simulink model "MoWiTO_mpc_FAST"  (Simulink 10.0)
settings: Solver=ode4  StartTime=0.0  StopTime=TMax  FixedStep=DT  MaxStep=DT  RelTol=1e-3  EnableMultiTasking=on
undefined symbols (not defined in the file or in its folder): beta_min, DiscIntNeverNeededParam, DT_control, DT_hw, FBonly, mpc, N, N_delay, N_filt, Nominal, OutList, strmatch, TurbParams
libraries: dspbuff3 x1
settings Model: Creator=bjonkman  LastModifiedBy=tskib
settings DataIOCC: LimitDataPoints=on  SignalLoggingSaveFormat=ModelDataLogs  SaveOutput=off  SaveTime=off  SignalLoggingName=sigsOut
settings OptimizationCC: ExpressionDepthLimit=2147483647
settings DebuggingCC: SaveWithParameterizedLinksMsg=none  SignalResolutionControl=TryResolveAllWithWarning  MultiTaskDSMMsg=warning  MultiTaskCondExecSysMsg=none  FcnCallInpInsideContextMsg=warning  AllowSymbolicDim=off  StateNameClashWarn=warning
settings HardwareCC: TargetUnknown=on
settings GRTTargetCC: GeneratePreprocessorConditionals=Disable all
settings ConfigComp: CovExternalEMLEnable=off

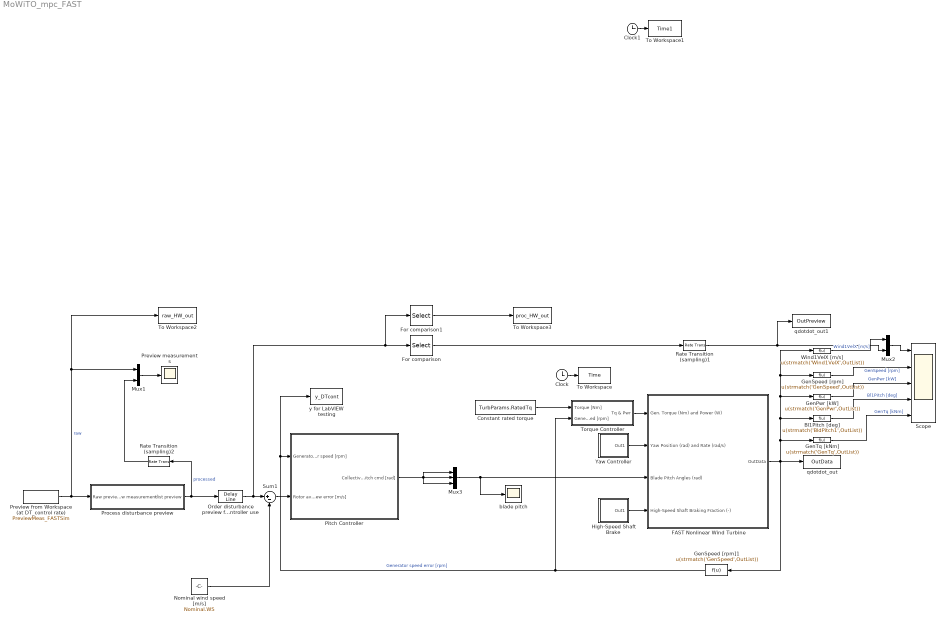
== system MoWiTO_mpc_FAST ==
  Bl1Pitch [deg] : Fcn  Expr=u(strmatch('BldPitch1',OutList))
  Clock : Clock
  Clock1 : Clock
  Constant rated torque : Constant  Value=TurbParams.RatedTq
  FAST Nonlinear Wind Turbine : Subsystem  mask(FAST Nonlinear Wind Turbine){}
      mask help: This block contains the FAST S-Function.
      mask init:
      | clear FAST_SFunc
  For comparison : Selector  InputPortWidth=N  IndexOptions=Index vector (dialog)  Indices=[1]  OutputSizes=1
  For comparison1 : Selector  InputPortWidth=N  IndexOptions=Index vector (dialog)  Indices=[N]  OutputSizes=1
  GenPwr [kW] : Fcn  Expr=u(strmatch('GenPwr',OutList))
  GenSpeed [rpm] : Fcn  Expr=u(strmatch('GenSpeed',OutList))
  GenSpeed [rpm]1 : Fcn  Expr=u(strmatch('GenSpeed',OutList))
  GenTq [kNm] : Fcn  Expr=u(strmatch('GenTq',OutList))
  High-Speed Shaft Brake : Subsystem
  Mux1 : Mux  Inputs=2
  Mux2 : Mux  Inputs=2
  Mux3 : Mux  Inputs=3
  Nominal wind speed [m/s] : Constant  Value=Nominal.WS
  Order disturbance preview for controller use : dspbuff3/Delay Line  siz=N  ic=Nominal.WS  directfeed=off  enable_output=off  hold_output=off  OutputFrames=off
      settings: SourceProductName=DSP System Toolbox  SourceProductBaseCode=DS
  Pitch Controller : Subsystem
  Preview from Workspace (at DT_control rate) : FromWorkspace  VariableName=PreviewMeas_FASTSim  SampleTime=DT_hw
  Preview measurements : Scope
  Process disturbance preview : Subsystem
  Rate Transition (sampling)1 : RateTransition  InitialCondition=Nominal.WS  OutPortSampleTime=DT
  Rate Transition (sampling)2 : RateTransition  OutPortSampleTime=DT_hw
  Scope : Scope  NumInputPorts=5
  Sum1 : Sum  Inputs=|+-
  To Workspace : ToWorkspace  VariableName=Time  SampleTime=-1
  To Workspace1 : ToWorkspace  VariableName=Time1  SampleTime=-1
  To Workspace2 : ToWorkspace  VariableName=raw_HW_out  SampleTime=-1
  To Workspace3 : ToWorkspace  VariableName=proc_HW_out  SampleTime=-1
  Torque Controller : Subsystem
  Wind1VelX [m/s] : Fcn  Expr=u(strmatch('Wind1VelX',OutList))
  Yaw Controller : Subsystem
  blade pitch : Scope
  qdotdot_out : ToWorkspace  VariableName=OutData  SampleTime=-1
  qdotdot_out1 : ToWorkspace  VariableName=OutPreview  SampleTime=-1
  y for LabVIEW testing : ToWorkspace  VariableName=y_DTcont  SampleTime=-1
  wires:
  Clock/1 -> To Workspace/1
  FAST Nonlinear Wind Turbine/1(OutData) -> GenSpeed [rpm]1/1, GenTq [kNm]/1, Bl1Pitch [deg]/1, GenPwr [kW]/1, GenSpeed [rpm]/1, Wind1VelX [m/s]/1, qdotdot_out/1
  Torque Controller/1(Tq & Pwr) -> FAST Nonlinear Wind Turbine/1(Gen. Torque (Nm) and Power (W))
  Yaw Controller/1(Out1) -> FAST Nonlinear Wind Turbine/2(Yaw Position (rad) and Rate (rad/s))
  Mux3/1 -> FAST Nonlinear Wind Turbine/3(Blade Pitch Angles (rad)), blade pitch/1
  High-Speed Shaft Brake/1(Out1) -> FAST Nonlinear Wind Turbine/4(High-Speed Shaft Braking Fraction (-))
  Constant rated torque/1 -> Torque Controller/1(Torque [Nm])
  Wind1VelX [m/s]/1 -> Mux2/1  "Wind1VelX [m/s]"
  GenSpeed [rpm]/1 -> Scope/2  "GenSpeed [rpm]"
  GenPwr [kW]/1 -> Scope/3  "GenPwr [kW]"
  Bl1Pitch [deg]/1 -> Scope/4  "Bl1Pitch [deg]"
  GenTq [kNm]/1 -> Scope/5  "GenTq [kNm]"
  GenSpeed [rpm]1/1 -> y for LabVIEW testing/1, Pitch Controller/1("Generator speed [rpm] "), Torque Controller/2(Generator speed [rpm])  "Generator speed error [rpm]"
  Process disturbance preview/1(dist preview) -> Order disturbance preview for controller use/1, Rate Transition (sampling)2/1  "processed"
  Clock1/1 -> To Workspace1/1
  Sum1/1 -> Pitch Controller/2(Rotor average speed preview error [m/s])
  Nominal wind speed [m/s]/1 -> Sum1/2
  Mux1/1 -> Preview measurements/1
  Preview from Workspace (at DT_control rate)/1 -> Process disturbance preview/1(Raw preview measurement), To Workspace2/1, Mux1/1  "raw"
  Mux2/1 -> Scope/1
  For comparison/1 -> Rate Transition (sampling)1/1
  Rate Transition (sampling)2/1 -> Mux1/2
  Rate Transition (sampling)1/1 -> qdotdot_out1/1, Mux2/2
  Pitch Controller/1(Collective pitch cmd [rad]) -> Mux3/3, Mux3/1, Mux3/2
  For comparison1/1 -> To Workspace3/1
  Order disturbance preview for controller use/1 -> For comparison1/1, For comparison/1, Sum1/1

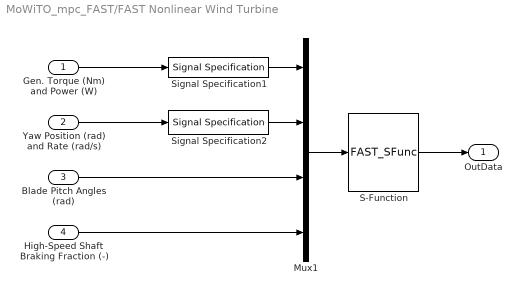
== system MoWiTO_mpc_FAST/FAST Nonlinear Wind Turbine ==
  Gen. Torque (Nm) and Power (W) : Inport
  Yaw Position (rad) and Rate (rad/s) : Inport  Port=2
  Blade Pitch Angles (rad) : Inport  Port=3
  High-Speed Shaft Braking Fraction (-) : Inport  Port=4
  Mux1 : Mux
  S-Function : S-Function  FunctionName=FAST_SFunc  Parameters=FAST_InputFileName, TMax, 0  SFunctionDeploymentMode=off  EnableBusSupport=off
  Signal Specification1 : SignalSpecification  OutDataTypeStr=double  Dimensions=2
  Signal Specification2 : SignalSpecification  OutDataTypeStr=double  Dimensions=2
  OutData : Outport
  wires:
  Gen. Torque (Nm) and Power (W)/1 -> Signal Specification1/1
  S-Function/1 -> OutData/1
  Mux1/1 -> S-Function/1
  Blade Pitch Angles (rad)/1 -> Mux1/3
  Yaw Position (rad) and Rate (rad/s)/1 -> Signal Specification2/1
  Signal Specification1/1 -> Mux1/1
  Signal Specification2/1 -> Mux1/2
  High-Speed Shaft Braking Fraction (-)/1 -> Mux1/4

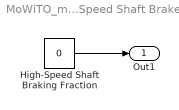
== system MoWiTO_mpc_FAST/High-Speed Shaft Brake ==
  High-Speed Shaft Braking Fraction : Constant  Value=0
  Out1 : Outport
  wires:
  High-Speed Shaft Braking Fraction/1 -> Out1/1

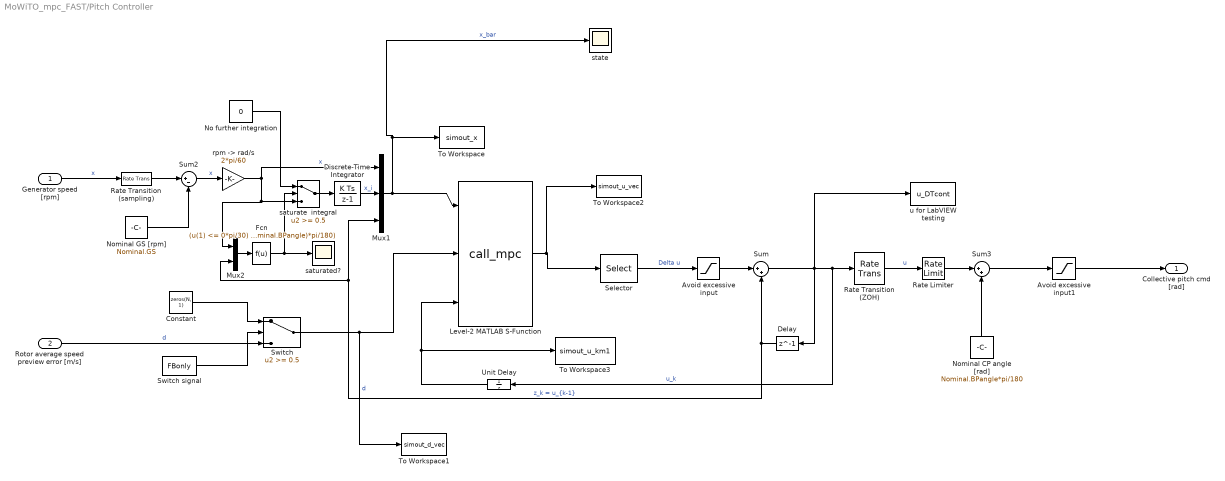
== system MoWiTO_mpc_FAST/Pitch Controller ==
  "Generator speed [rpm] " : Inport
  Rotor average speed preview error [m/s] : Inport  Port=2
  Avoid excessive input : Saturate  UpperLimit=TurbParams.PitchRateLimit*DT_control  LowerLimit=-TurbParams.PitchRateLimit*DT_control
  Avoid excessive input1 : Saturate  UpperLimit=inf  LowerLimit=beta_min*pi/180
  Constant : Constant  Value=zeros(N, 1)
  Delay : Delay  DelayLength=1  InitialCondition=0  SampleTime=DT_control
  Discrete-Time Integrator : DiscreteIntegrator  SampleTime=DT_control  ICPrevOutput=DiscIntNeverNeededParam  ICPrevScaledInput=DiscIntNeverNeededParam
  Fcn : Fcn  Expr=(u(1) <= 0*pi/30) && (u(2) <= (beta_min - Nominal.BPangle)*pi/180)
  Level-2 MATLAB S-Function : M-S-Function  FunctionName=call_mpc  Parameters=mpc
  Mux1 : Mux  Inputs=3
  Mux2 : Mux  Inputs=2
  No further integration : Constant  Value=0
  Nominal CP angle [rad] : Constant  Value=Nominal.BPangle*pi/180
  Nominal GS [rpm] : Constant  Value=Nominal.GS
  Rate Limiter : RateLimiter  RisingSlewLimit=TurbParams.PitchRateLimit  FallingSlewLimit=-TurbParams.PitchRateLimit  SampleTimeMode=inherited
  Rate Transition (ZOH) : RateTransition  OutPortSampleTime=DT
  Rate Transition (sampling) : RateTransition  OutPortSampleTime=DT_control
  Selector : Selector  InputPortWidth=mpc.Mdl.m*mpc.N  IndexOptions=Index vector (dialog)  Indices=[1:mpc.Mdl.m]  OutputSizes=1
  Sum : Sum  Inputs=|++  OutDataTypeStr=Inherit: Inherit via back propagation
  Sum2 : Sum  Inputs=|+-
  Sum3 : Sum  Inputs=|++
  Switch : Switch  Threshold=0.5
  Switch signal : Constant  Value=FBonly
  To Workspace : ToWorkspace  VariableName=simout_x  SampleTime=-1
  To Workspace1 : ToWorkspace  VariableName=simout_d_vec  SampleTime=-1
  To Workspace2 : ToWorkspace  VariableName=simout_u_vec  SampleTime=-1
  To Workspace3 : ToWorkspace  VariableName=simout_u_km1  SampleTime=-1
  Unit Delay : UnitDelay  SampleTime=DT_control  HasFrameUpgradeWarning=on
  "rpm -> rad/s" : Gain  Gain=2*pi/60
  saturate  integral : Switch  Threshold=0.5
  saturated? : Scope
  state : Scope
  u for LabVIEW testing : ToWorkspace  VariableName=u_DTcont  SampleTime=-1
  Collective pitch cmd [rad] : Outport
  wires:
  Delay/1 -> Mux1/3, Mux2/2, Sum/2  "z_k = u_{k-1}"
  Sum/1 -> u for LabVIEW testing/1, Unit Delay/1, Rate Transition (ZOH)/1, Delay/1  "u_k"
  Selector/1 -> Avoid excessive input/1  "Delta u"
  Rotor average speed preview error [m/s]/1 -> Switch/3  "d"
  "rpm -> rad/s"/1 -> Mux2/1, saturate  integral/3, Mux1/1  "x"
  Discrete-Time Integrator/1 -> Mux1/2  "x_i"
  Sum2/1 -> "rpm -> rad/s"/1  "x"
  Mux1/1 -> state/1, To Workspace/1, Level-2 MATLAB S-Function/1  "x_bar"
  Avoid excessive input/1 -> Sum/1
  Nominal GS [rpm]/1 -> Sum2/2
  "Generator speed [rpm] "/1 -> Rate Transition (sampling)/1  "x"
  Rate Transition (sampling)/1 -> Sum2/1
  Nominal CP angle [rad]/1 -> Sum3/2
  Rate Limiter/1 -> Sum3/1
  Rate Transition (ZOH)/1 -> Rate Limiter/1  "u"
  Switch signal/1 -> Switch/2
  Level-2 MATLAB S-Function/1 -> To Workspace2/1, Selector/1
  Sum3/1 -> Avoid excessive input1/1
  Unit Delay/1 -> Level-2 MATLAB S-Function/3, To Workspace3/1
  Switch/1 -> Level-2 MATLAB S-Function/2, To Workspace1/1  "d"
  Constant/1 -> Switch/1
  Avoid excessive input1/1 -> Collective pitch cmd [rad]/1
  saturate  integral/1 -> Discrete-Time Integrator/1
  No further integration/1 -> saturate  integral/1
  Mux2/1 -> Fcn/1
  Fcn/1 -> saturated?/1, saturate  integral/2

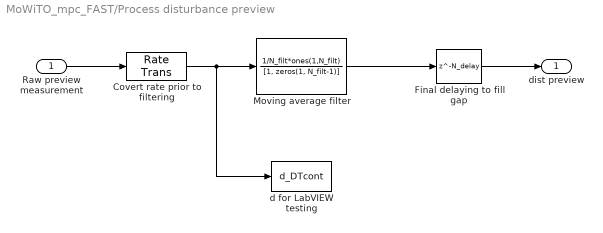
== system MoWiTO_mpc_FAST/Process disturbance preview ==
  Raw preview measurement : Inport
  "Covert rate prior to filtering " : RateTransition  InitialCondition=Nominal.WS  OutPortSampleTime=DT_control
  Final delaying to fill gap : Delay  DelayLength=N_delay  InitialCondition=Nominal.WS*ones(1, N_delay)  SampleTime=DT_control
  Moving average filter : DiscreteTransferFcn  Numerator=1/N_filt*ones(1,N_filt)  Denominator=[1, zeros(1, N_filt-1)]  InitialStates=Nominal.WS*ones(N_filt-1, 1)  SampleTime=DT_control
  d for LabVIEW testing : ToWorkspace  VariableName=d_DTcont  SampleTime=-1
  dist preview : Outport
  wires:
  Raw preview measurement/1 -> "Covert rate prior to filtering "/1
  Final delaying to fill gap/1 -> dist preview/1
  Moving average filter/1 -> Final delaying to fill gap/1
  "Covert rate prior to filtering "/1 -> d for LabVIEW testing/1, Moving average filter/1

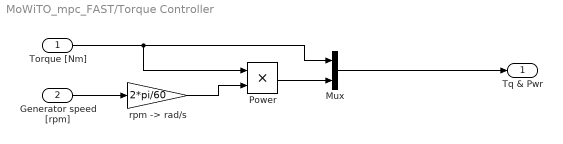
== system MoWiTO_mpc_FAST/Torque Controller ==
  Torque [Nm] : Inport
  Generator speed [rpm] : Inport  Port=2
  Mux : Mux  Inputs=2
  Power : Product
  "rpm -> rad/s" : Gain  Gain=2*pi/60
  Tq & Pwr : Outport
  wires:
  Mux/1 -> Tq & Pwr/1
  Torque [Nm]/1 -> Power/1, Mux/1
  Power/1 -> Mux/2
  Generator speed [rpm]/1 -> "rpm -> rad/s"/1
  "rpm -> rad/s"/1 -> Power/2

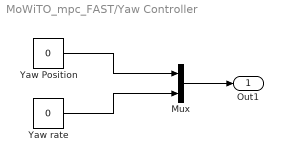
== system MoWiTO_mpc_FAST/Yaw Controller ==
  Mux : Mux  Inputs=2
  Yaw Position : Constant  Value=0
  Yaw rate : Constant  Value=0
  Out1 : Outport
  wires:
  Mux/1 -> Out1/1
  Yaw Position/1 -> Mux/1
  Yaw rate/1 -> Mux/2
